simulink model "greenhouse_final"  (R2026a)
settings: Solver=FixedStepAuto  StopTime=86400  FixedStep=Ts
values from neighbouring files (symbols this model uses):
  a_RH = 0.02    [greenhouse_parameters.m]
  a_S = 0.5    [greenhouse_parameters.m]
  a_T = 0.04    [greenhouse_parameters.m]
  C_T = 1000    [greenhouse_parameters.m]
  E0 = 0.0000833    (= 8.33e-05)    [greenhouse_parameters.m]
  K_fan = 0.30    (= 0.3)    [greenhouse_parameters.m]
  K_heater = 1.0    (= 1)    [greenhouse_parameters.m]
  K_humidity = 0.0005    [greenhouse_parameters.m]
  K_irrigation = 0.003    [greenhouse_parameters.m]
  K_loss = 0.20    (= 0.2)    [greenhouse_parameters.m]
  K_pump = 0.001    [greenhouse_parameters.m]
  K_solar = 0.001    [greenhouse_parameters.m]
  K_vent = 0.001    [greenhouse_parameters.m]
  M0 = 42    [generate_training_data.m]    (also in greenhouse_parameters.m = 50; run_all_scenarios.m = 45)
  mu_fan = [28.1915532245 66.9272905065 0.767464723572]    [AI_train_test_data_v4.mat]    (also in greenhouse_AI_models_v4.mat; prepare_ai_dataset.m = mean(X_fan_train,1))
  mu_heater = [28.1915532245 0.168979875087]    [AI_train_test_data_v4.mat]    (also in greenhouse_AI_models_v4.mat; prepare_ai_dataset.m = mean(X_heater_train,1))
  mu_pump = [51.2258877908 0.0955355077492]    [AI_train_test_data_v4.mat]    (also in greenhouse_AI_models_v4.mat; prepare_ai_dataset.m = mean(X_pump_train,1))
  RH0 = 65    [generate_training_data.m]    (also in greenhouse_parameters.m = 60; run_all_scenarios.m = 55)
  RH_amp = 15    [generate_training_data.m]    (also in greenhouse_parameters.m = 10; run_all_scenarios.m)
  RH_bias = 65    [generate_training_data.m]    (also in greenhouse_parameters.m = 70; run_all_scenarios.m = 55)
  sigma_fan = [5.94814277773 19.3183251688 0.422460581324]    [AI_train_test_data_v4.mat]    (also in greenhouse_AI_models_v4.mat; prepare_ai_dataset.m = std(X_fan_train,0,1))
  sigma_heater = [5.94814277773 0.374744977576]    [AI_train_test_data_v4.mat]    (also in greenhouse_AI_models_v4.mat; prepare_ai_dataset.m = std(X_heater_train,0,1))
  sigma_pump = [6.77959476992 0.293961684268]    [AI_train_test_data_v4.mat]    (also in greenhouse_AI_models_v4.mat; prepare_ai_dataset.m = std(X_pump_train,0,1))
  Solar_amp = 300    [generate_training_data.m]    (also in greenhouse_parameters.m = 500; run_all_scenarios.m = 350)
  Solar_bias = 550    [generate_training_data.m]    (also in greenhouse_parameters.m = 500; run_all_scenarios.m = 650)
  T0 = 24    [generate_training_data.m]    (also in greenhouse_parameters.m = 25; run_all_scenarios.m = 25)
  T_amp = 9    [generate_training_data.m]    (also in greenhouse_parameters.m = 7; run_all_scenarios.m = 7)
  T_bias = 24    [generate_training_data.m]    (also in greenhouse_parameters.m = 28; run_all_scenarios.m = 29)
  Ts = 60    [greenhouse_parameters.m]
libraries: statsLibrary x3
settings Model: Creator=Milan  LastModifiedBy=Milan

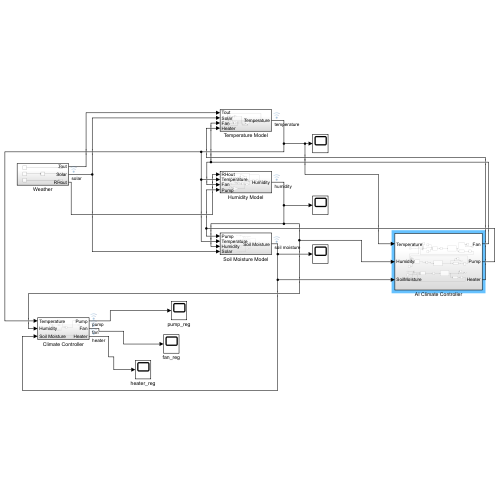
[thumbnail: Simulink's stored preview of the top-level diagram]
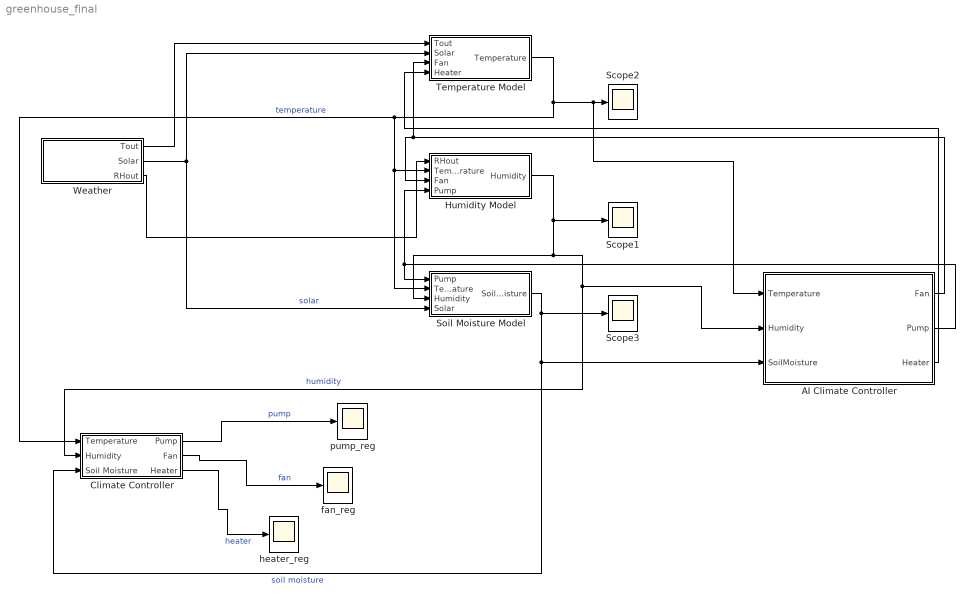
== system greenhouse_final ==
  AI Climate Controller : Subsystem
  Climate Controller : Subsystem
  Humidity Model : Subsystem
  Scope1 : Scope
      settings: ActiveDisplayYMinimum=36.510410481931025  ActiveDisplayYMaximum=74.5543246381449
  Scope2 : Scope
      settings: ActiveDisplayYMinimum=22.477962989488532  ActiveDisplayYMaximum=39.635587368258683
  Scope3 : Scope
      settings: ActiveDisplayYMinimum=38.739539381371436  ActiveDisplayYMaximum=51.2749472709106  DataLoggingVariableName=ScopeData2
  Soil Moisture Model : Subsystem
  Temperature Model : Subsystem
  Weather : Subsystem
  fan_reg : Scope
      settings: ActiveDisplayYMinimum=-0.12499999999999997  ActiveDisplayYMaximum=1.125  DataLoggingVariableName=ScopeData4
  heater_reg : Scope
      settings: ActiveDisplayYMinimum=-1  ActiveDisplayYMaximum=1  DataLoggingVariableName=ScopeData5
  pump_reg : Scope
      settings: ActiveDisplayYMinimum=-0.12499999999999997  ActiveDisplayYMaximum=1.125  DataLoggingVariableName=ScopeData3
  wires:
  Weather/2(Solar) -> Soil Moisture Model/4(Solar), Temperature Model/2(Solar)  "solar"
  Weather/1(Tout) -> Temperature Model/1(Tout)
  Weather/3(RHout) -> Humidity Model/1(RHout)
  Temperature Model/1(Temperature) -> AI Climate Controller/1(Temperature), Scope2/1, Climate Controller/1(Temperature), Soil Moisture Model/2(Temperature), Humidity Model/2(Temperature)  "temperature"
  Humidity Model/1(Humidity) -> Soil Moisture Model/3(Humidity), Climate Controller/2(Humidity), AI Climate Controller/2(Humidity), Scope1/1  "humidity"
  Soil Moisture Model/1(Soil Moisture) -> AI Climate Controller/3(SoilMoisture), Climate Controller/3(Soil Moisture), Scope3/1  "soil moisture"
  Climate Controller/1(Pump) -> pump_reg/1  "pump"
  Climate Controller/2(Fan) -> fan_reg/1  "fan"
  Climate Controller/3(Heater) -> heater_reg/1  "heater"
  AI Climate Controller/1(Fan) -> Humidity Model/3(Fan), Temperature Model/3(Fan)
  AI Climate Controller/2(Pump) -> Humidity Model/4(Pump), Soil Moisture Model/1(Pump)
  AI Climate Controller/3(Heater) -> Temperature Model/4(Heater)

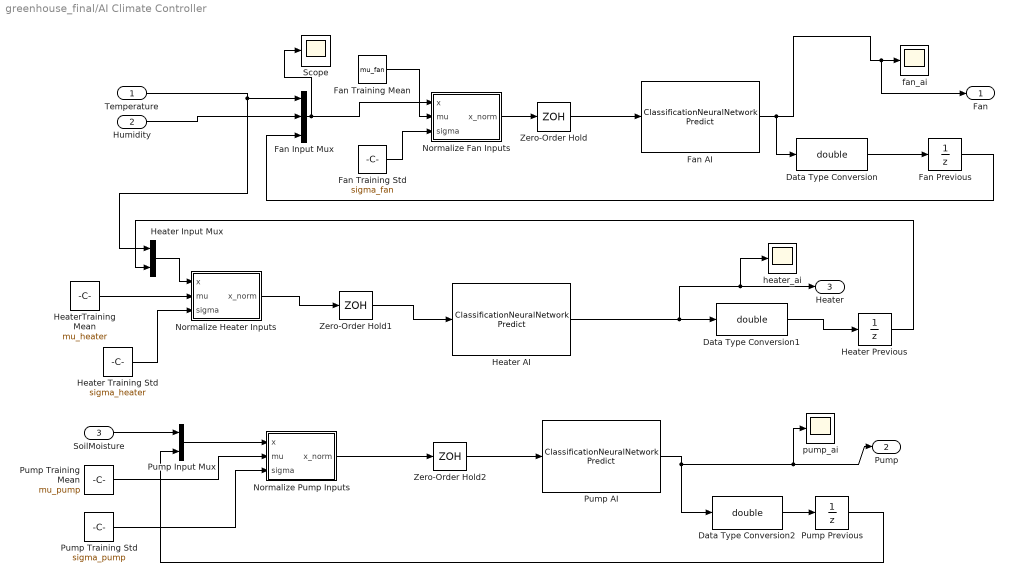
== system greenhouse_final/AI Climate Controller ==
  Temperature : Inport
  Humidity : Inport  Port=2
  SoilMoisture : Inport  Port=3
  Data Type Conversion : DataTypeConversion  OutDataTypeStr=double  SaturateOnIntegerOverflow=off  RndMeth=Floor
  Data Type Conversion1 : DataTypeConversion  OutDataTypeStr=double  SaturateOnIntegerOverflow=off  RndMeth=Floor
  Data Type Conversion2 : DataTypeConversion  OutDataTypeStr=double  SaturateOnIntegerOverflow=off  RndMeth=Floor
  Fan AI : statsLibrary/Classification/ClassificationNeuralNetwork Predict  TrainedLearner=fanModel  ShowOutputScore=off  LabelDataTypeStr=Inherit: Inherit via back propagation  LabelOutMin=[]  LabelOutMax=[]  ScoreOutMin=[]  ScoreOutMax=[]  RawScoreOutMin=[]  RawScoreOutMax=[]  OutputLayerOutMin=[]  OutputLayerOutMax=[]  OutputLayerAdditionOutMin=[]  OutputLayerAdditionOutMax=[]  LayerSelector=Layer 1  Layer1OutMin=[]  Layer1OutMax=[]  Layer1AdditionOutMin=[]  Layer1AdditionOutMax=[]  Layer2OutMin=[]  Layer2OutMax=[]  Layer2AdditionOutMin=[]  Layer2AdditionOutMax=[]  Layer3OutMin=[]  Layer3OutMax=[]  Layer3AdditionOutMin=[]  Layer3AdditionOutMax=[]  Layer4OutMin=[]  Layer4OutMax=[]  Layer4AdditionOutMin=[]  Layer4AdditionOutMax=[]  Layer5OutMin=[]  Layer5OutMax=[]  Layer5AdditionOutMin=[]  Layer5AdditionOutMax=[]  Layer6OutMin=[]  Layer6OutMax=[]  Layer6AdditionOutMin=[]  Layer6AdditionOutMax=[]  Layer7OutMin=[]  Layer7OutMax=[]  Layer7AdditionOutMin=[]  Layer7AdditionOutMax=[]  Layer8OutMin=[]  Layer8OutMax=[]  Layer8AdditionOutMin=[]  Layer8AdditionOutMax=[]  Layer9OutMin=[]  Layer9OutMax=[]  Layer9AdditionOutMin=[]  Layer9AdditionOutMax=[]  Layer10OutMin=[]  Layer10OutMax=[]  Layer10AdditionOutMin=[]  Layer10AdditionOutMax=[]  Layer11OutMin=[]  Layer11OutMax=[]  Layer11AdditionOutMin=[]  Layer11AdditionOutMax=[]  SoftmaxSumOutMin=[]  SoftmaxSumOutMax=[]  SoftmaxDiffOutMin=[]  SoftmaxDiffOutMax=[]  StandardizedInputOutMin=[]  StandardizedInputOutMax=[]  StoredEnumName=treeMdl_enumLabels  NumHiddenLayers=1
  Fan Input Mux : Mux  Inputs=3
  Fan Previous : UnitDelay  SampleTime=Ts
  Fan Training Mean : Constant  Value=mu_fan
  Fan Training Std : Constant  Value=sigma_fan
  Heater AI : statsLibrary/Classification/ClassificationNeuralNetwork Predict  TrainedLearner=heaterModel  ShowOutputScore=off  LabelDataTypeStr=Inherit: Inherit via back propagation  LabelOutMin=[]  LabelOutMax=[]  ScoreOutMin=[]  ScoreOutMax=[]  RawScoreOutMin=[]  RawScoreOutMax=[]  OutputLayerOutMin=[]  OutputLayerOutMax=[]  OutputLayerAdditionOutMin=[]  OutputLayerAdditionOutMax=[]  LayerSelector=Layer 1  Layer1OutMin=[]  Layer1OutMax=[]  Layer1AdditionOutMin=[]  Layer1AdditionOutMax=[]  Layer2OutMin=[]  Layer2OutMax=[]  Layer2AdditionOutMin=[]  Layer2AdditionOutMax=[]  Layer3OutMin=[]  Layer3OutMax=[]  Layer3AdditionOutMin=[]  Layer3AdditionOutMax=[]  Layer4OutMin=[]  Layer4OutMax=[]  Layer4AdditionOutMin=[]  Layer4AdditionOutMax=[]  Layer5OutMin=[]  Layer5OutMax=[]  Layer5AdditionOutMin=[]  Layer5AdditionOutMax=[]  Layer6OutMin=[]  Layer6OutMax=[]  Layer6AdditionOutMin=[]  Layer6AdditionOutMax=[]  Layer7OutMin=[]  Layer7OutMax=[]  Layer7AdditionOutMin=[]  Layer7AdditionOutMax=[]  Layer8OutMin=[]  Layer8OutMax=[]  Layer8AdditionOutMin=[]  Layer8AdditionOutMax=[]  Layer9OutMin=[]  Layer9OutMax=[]  Layer9AdditionOutMin=[]  Layer9AdditionOutMax=[]  Layer10OutMin=[]  Layer10OutMax=[]  Layer10AdditionOutMin=[]  Layer10AdditionOutMax=[]  Layer11OutMin=[]  Layer11OutMax=[]  Layer11AdditionOutMin=[]  Layer11AdditionOutMax=[]  SoftmaxSumOutMin=[]  SoftmaxSumOutMax=[]  SoftmaxDiffOutMin=[]  SoftmaxDiffOutMax=[]  StandardizedInputOutMin=[]  StandardizedInputOutMax=[]  StoredEnumName=treeMdl_enumLabels  NumHiddenLayers=1
  Heater Input Mux : Mux  Inputs=2
  Heater Previous : UnitDelay  SampleTime=Ts
  Heater Training Std : Constant  Value=sigma_heater
  HeaterTraining Mean : Constant  Value=mu_heater
  Normalize Fan Inputs : MATLAB Function  TreatAsAtomicUnit=on
  Normalize Heater Inputs : MATLAB Function  TreatAsAtomicUnit=on
  Normalize Pump Inputs : MATLAB Function  TreatAsAtomicUnit=on
  Pump AI : statsLibrary/Classification/ClassificationNeuralNetwork Predict  TrainedLearner=pumpModel  ShowOutputScore=off  LabelDataTypeStr=Inherit: Inherit via back propagation  LabelOutMin=[]  LabelOutMax=[]  ScoreOutMin=[]  ScoreOutMax=[]  RawScoreOutMin=[]  RawScoreOutMax=[]  OutputLayerOutMin=[]  OutputLayerOutMax=[]  OutputLayerAdditionOutMin=[]  OutputLayerAdditionOutMax=[]  LayerSelector=Layer 1  Layer1OutMin=[]  Layer1OutMax=[]  Layer1AdditionOutMin=[]  Layer1AdditionOutMax=[]  Layer2OutMin=[]  Layer2OutMax=[]  Layer2AdditionOutMin=[]  Layer2AdditionOutMax=[]  Layer3OutMin=[]  Layer3OutMax=[]  Layer3AdditionOutMin=[]  Layer3AdditionOutMax=[]  Layer4OutMin=[]  Layer4OutMax=[]  Layer4AdditionOutMin=[]  Layer4AdditionOutMax=[]  Layer5OutMin=[]  Layer5OutMax=[]  Layer5AdditionOutMin=[]  Layer5AdditionOutMax=[]  Layer6OutMin=[]  Layer6OutMax=[]  Layer6AdditionOutMin=[]  Layer6AdditionOutMax=[]  Layer7OutMin=[]  Layer7OutMax=[]  Layer7AdditionOutMin=[]  Layer7AdditionOutMax=[]  Layer8OutMin=[]  Layer8OutMax=[]  Layer8AdditionOutMin=[]  Layer8AdditionOutMax=[]  Layer9OutMin=[]  Layer9OutMax=[]  Layer9AdditionOutMin=[]  Layer9AdditionOutMax=[]  Layer10OutMin=[]  Layer10OutMax=[]  Layer10AdditionOutMin=[]  Layer10AdditionOutMax=[]  Layer11OutMin=[]  Layer11OutMax=[]  Layer11AdditionOutMin=[]  Layer11AdditionOutMax=[]  SoftmaxSumOutMin=[]  SoftmaxSumOutMax=[]  SoftmaxDiffOutMin=[]  SoftmaxDiffOutMax=[]  StandardizedInputOutMin=[]  StandardizedInputOutMax=[]  StoredEnumName=treeMdl_enumLabels  NumHiddenLayers=1
  Pump Input Mux : Mux  Inputs=2
  Pump Previous : UnitDelay  SampleTime=Ts
  Pump Training Mean : Constant  Value=mu_pump
  Pump Training Std : Constant  Value=sigma_pump
  Scope : Scope
      settings: ActiveDisplayYMinimum=-31.25  ActiveDisplayYMaximum=281.25000000000006  DataLoggingVariableName=ScopeData9
  Zero-Order Hold : ZeroOrderHold  SampleTime=Ts
  Zero-Order Hold1 : ZeroOrderHold  SampleTime=Ts
  Zero-Order Hold2 : ZeroOrderHold  SampleTime=Ts
  fan_ai : Scope
      settings: ActiveDisplayYMinimum=-0.12499999999999997  ActiveDisplayYMaximum=1.125  DataLoggingVariableName=ScopeData6
  heater_ai : Scope
      settings: ActiveDisplayYMinimum=-1  ActiveDisplayYMaximum=1  DataLoggingVariableName=ScopeData7
  pump_ai : Scope
      settings: ActiveDisplayYMinimum=-0.12499999999999997  ActiveDisplayYMaximum=1.125  DataLoggingVariableName=ScopeData8
  Fan : Outport
  Pump : Outport  Port=2
  Heater : Outport  Port=3
  wires:
  Fan AI/1 -> Data Type Conversion/1, Fan/1, fan_ai/1
  Humidity/1 -> Fan Input Mux/2
  Temperature/1 -> Heater Input Mux/1, Fan Input Mux/1
  SoilMoisture/1 -> Pump Input Mux/1
  Normalize Heater Inputs/1(x_norm) -> Zero-Order Hold1/1
  Heater AI/1 -> Data Type Conversion1/1, heater_ai/1, Heater/1
  Pump AI/1 -> Data Type Conversion2/1, pump_ai/1, Pump/1
  Data Type Conversion/1 -> Fan Previous/1
  Data Type Conversion1/1 -> Heater Previous/1
  Data Type Conversion2/1 -> Pump Previous/1
  Pump Previous/1 -> Pump Input Mux/2
  Pump Training Mean/1 -> Normalize Pump Inputs/2(mu)
  Pump Input Mux/1 -> Normalize Pump Inputs/1(x)
  Pump Training Std/1 -> Normalize Pump Inputs/3(sigma)
  Normalize Pump Inputs/1(x_norm) -> Zero-Order Hold2/1
  Fan Previous/1 -> Fan Input Mux/3
  Fan Input Mux/1 -> Scope/1, Normalize Fan Inputs/1(x)
  Fan Training Mean/1 -> Normalize Fan Inputs/2(mu)
  Fan Training Std/1 -> Normalize Fan Inputs/3(sigma)
  Heater Previous/1 -> Heater Input Mux/2
  Normalize Fan Inputs/1(x_norm) -> Zero-Order Hold/1
  Heater Input Mux/1 -> Normalize Heater Inputs/1(x)
  HeaterTraining Mean/1 -> Normalize Heater Inputs/2(mu)
  Heater Training Std/1 -> Normalize Heater Inputs/3(sigma)
  Zero-Order Hold/1 -> Fan AI/1
  Zero-Order Hold1/1 -> Heater AI/1
  Zero-Order Hold2/1 -> Pump AI/1

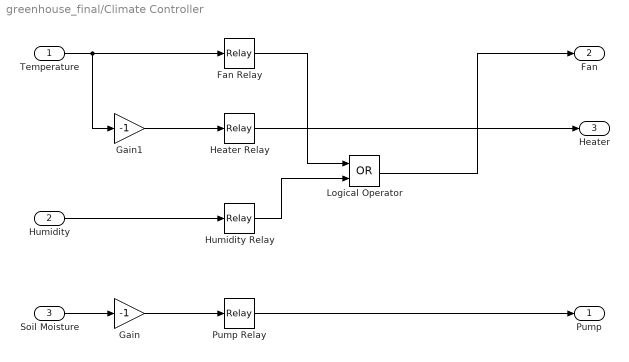
== system greenhouse_final/Climate Controller ==
  Temperature : Inport
  Humidity : Inport  Port=2
  Soil Moisture : Inport  Port=3
  Fan Relay : Relay  OnSwitchValue=30  OffSwitchValue=28
  Gain : Gain  Gain=-1
  Gain1 : Gain  Gain=-1
  Heater Relay : Relay  OnSwitchValue=-22  OffSwitchValue=-24
  Humidity Relay : Relay  OnSwitchValue=80  OffSwitchValue=75
  Logical Operator : Logic  Operator=OR  AllPortsSameDT=off  OutDataTypeStr=boolean
  Pump Relay : Relay  OnSwitchValue=-40  OffSwitchValue=-50
  Pump : Outport
  Fan : Outport  Port=2
  Heater : Outport  Port=3
  wires:
  Soil Moisture/1 -> Gain/1
  Gain/1 -> Pump Relay/1
  Pump Relay/1 -> Pump/1
  Temperature/1 -> Gain1/1, Fan Relay/1
  Heater Relay/1 -> Heater/1
  Gain1/1 -> Heater Relay/1
  Humidity/1 -> Humidity Relay/1
  Fan Relay/1 -> Logical Operator/1
  Humidity Relay/1 -> Logical Operator/2
  Logical Operator/1 -> Fan/1

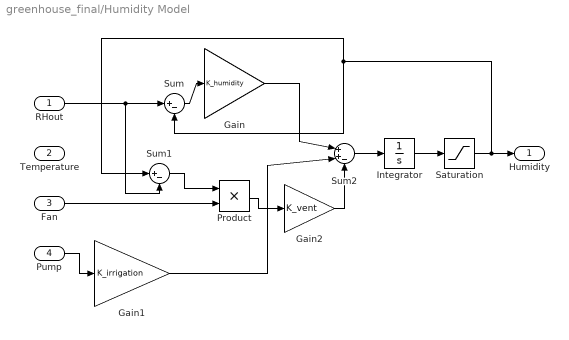
== system greenhouse_final/Humidity Model ==
  RHout : Inport
  Temperature : Inport  Port=2
  Fan : Inport  Port=3
  Pump : Inport  Port=4
  Gain : Gain  Gain=K_humidity
  Gain1 : Gain  Gain=K_irrigation
  Gain2 : Gain  Gain=K_vent
  Integrator : Integrator  InitialCondition=RH0
  Product : Product
  Saturation : Saturate  UpperLimit=100  LowerLimit=0
  Sum : Sum  Inputs=|+-
  Sum1 : Sum  Inputs=|+-
  Sum2 : Sum  Inputs=|++-
  Humidity : Outport
  wires:
  RHout/1 -> Sum1/2, Sum/1
  Sum/1 -> Gain/1
  Pump/1 -> Gain1/1
  Sum1/1 -> Product/1
  Fan/1 -> Product/2
  Product/1 -> Gain2/1
  Gain/1 -> Sum2/1
  Gain1/1 -> Sum2/2
  Gain2/1 -> Sum2/3
  Sum2/1 -> Integrator/1
  Integrator/1 -> Saturation/1
  Saturation/1 -> Sum1/1, Sum/2, Humidity/1

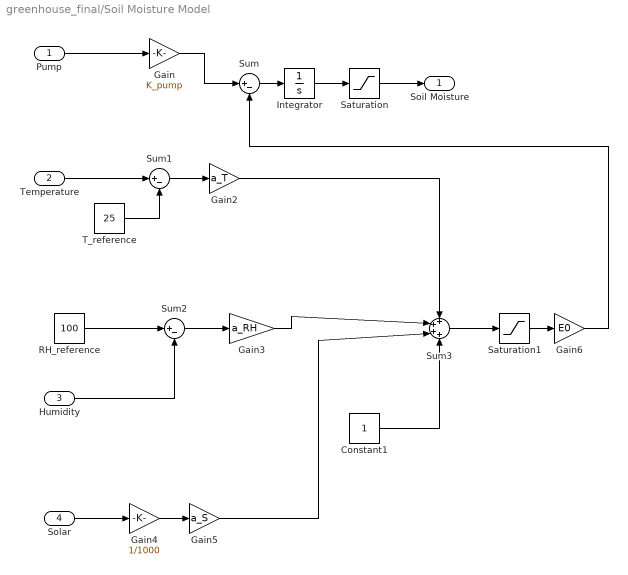
== system greenhouse_final/Soil Moisture Model ==
  Pump : Inport
  Temperature : Inport  Port=2
  Humidity : Inport  Port=3
  Solar : Inport  Port=4
  Constant1 : Constant
  Gain : Gain  Gain=K_pump
  Gain2 : Gain  Gain=a_T
  Gain3 : Gain  Gain=a_RH
  Gain4 : Gain  Gain=1/1000
  Gain5 : Gain  Gain=a_S
  Gain6 : Gain  Gain=E0
  Integrator : Integrator  InitialCondition=M0
  RH_reference : Constant  Value=100
  Saturation : Saturate  UpperLimit=100  LowerLimit=0
  Saturation1 : Saturate  UpperLimit=10  LowerLimit=0
  Sum : Sum  Inputs=|+-
  Sum1 : Sum  Inputs=|+-
  Sum2 : Sum  Inputs=|+-
  Sum3 : Sum  Inputs=++++
  T_reference : Constant  Value=25
  Soil Moisture : Outport
  wires:
  Pump/1 -> Gain/1
  Gain/1 -> Sum/1
  Sum/1 -> Integrator/1
  Integrator/1 -> Saturation/1
  Saturation/1 -> Soil Moisture/1
  Temperature/1 -> Sum1/1
  T_reference/1 -> Sum1/2
  Sum1/1 -> Gain2/1
  RH_reference/1 -> Sum2/1
  Humidity/1 -> Sum2/2
  Sum2/1 -> Gain3/1
  Solar/1 -> Gain4/1
  Gain4/1 -> Gain5/1
  Gain2/1 -> Sum3/1
  Gain3/1 -> Sum3/2
  Gain5/1 -> Sum3/3
  Constant1/1 -> Sum3/4
  Sum3/1 -> Saturation1/1
  Saturation1/1 -> Gain6/1
  Gain6/1 -> Sum/2

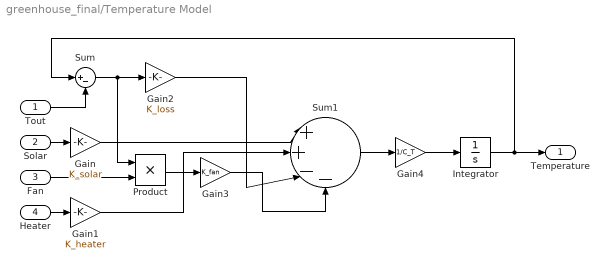
== system greenhouse_final/Temperature Model ==
  Tout : Inport
  Solar : Inport  Port=2
  Fan : Inport  Port=3
  Heater : Inport  Port=4
  Gain : Gain  Gain=K_solar
  Gain1 : Gain  Gain=K_heater
  Gain2 : Gain  Gain=K_loss
  Gain3 : Gain  Gain=K_fan
  Gain4 : Gain  Gain=1/C_T
  Integrator : Integrator  InitialCondition=T0
  Product : Product
  Sum : Sum  Inputs=|+-
  Sum1 : Sum  Inputs=|++--
  Temperature : Outport
  wires:
  Solar/1 -> Gain/1
  Heater/1 -> Gain1/1
  Tout/1 -> Sum/2
  Sum/1 -> Product/1, Gain2/1
  Fan/1 -> Product/2
  Product/1 -> Gain3/1
  Gain/1 -> Sum1/1
  Gain1/1 -> Sum1/2
  Gain3/1 -> Sum1/4
  Gain2/1 -> Sum1/3
  Sum1/1 -> Gain4/1
  Gain4/1 -> Integrator/1
  Integrator/1 -> Sum/1, Temperature/1

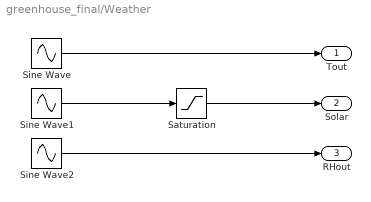
== system greenhouse_final/Weather ==
  Saturation : Saturate  UpperLimit=1000  LowerLimit=0
  Sine Wave : Sin  Amplitude=T_amp  Bias=T_bias  Frequency=2*pi/86400  Phase=-pi/2  SampleTime=Ts
  Sine Wave1 : Sin  Amplitude=Solar_amp  Bias=Solar_bias  Frequency=2*pi/86400  Phase=-pi/2  SampleTime=Ts
  Sine Wave2 : Sin  Amplitude=RH_amp  Bias=RH_bias  Frequency=2*pi/86400  Phase=-pi/2  SampleTime=Ts
  Tout : Outport
  Solar : Outport  Port=2
  RHout : Outport  Port=3
  wires:
  Sine Wave/1 -> Tout/1
  Sine Wave1/1 -> Saturation/1
  Saturation/1 -> Solar/1
  Sine Wave2/1 -> RHout/1

== matlab function greenhouse_final/AI Climate Controller/Normalize Heater Inputs ==
  data: x input; x_norm output; mu input; sigma input
function x_norm = fcn(x,mu,sigma)

x = x(:);
mu = mu(:);
sigma = sigma(:);

x_norm = (x - mu) ./ sigma;

end

== matlab function greenhouse_final/AI Climate Controller/Normalize Fan Inputs ==
  data: x input; x_norm output; mu input; sigma input
function x_norm = fcn(x,mu,sigma)

x = x(:);
mu = mu(:);
sigma = sigma(:);

x_norm = (x - mu) ./ sigma;

end

== matlab function greenhouse_final/AI Climate Controller/Normalize Pump Inputs ==
  data: x input; x_norm output; mu input; sigma input
function x_norm = fcn(x,mu,sigma)

x = x(:);
mu = mu(:);
sigma = sigma(:);

x_norm = (x - mu) ./ sigma;

end
